simulink model "Validity"  (R2021b)
settings: Solver=FixedStepDiscrete  StartTime=0.0  StopTime=10.0  FixedStep=0.1  RelTol=1e-3  EnableMultiTasking=on
undefined symbols (not defined in the file or in its folder): sldvsubsys
libraries: sldvlib x1
settings Model: DVExtractedSubsystem=Validity  Creator=Alessandro  LastModifiedBy=Alessandro
settings SolverCC: AlgebraicLoopSolver=TrustRegion  AutoInsertRateTranBlk=on
settings DataIOCC: LimitDataPoints=on
settings OptimizationCC: LifeSpan=inf
settings DebuggingCC: FrameProcessingCompatibilityMsg=none  AllowSymbolicDim=off  SFUnexpectedBacktrackingDiag=warning  SFNoUnconditionalDefaultTransitionDiag=warning  SFExecutionAtInitializationDiag=none  ArithmeticOperatorsInVariantConditions=warning
settings SFSimCC: SimUseLocalCustomCode=off  CustomCodeUndefinedFunction=UseInterfaceOnly
settings RTWCC: RTWUseLocalCustomCode=off
settings CodeAppCC: StateflowObjectComments=on
settings GRTTargetCC: TargetLangStandard=C89/C90 (ANSI)
settings ConfigComp: CovMetricSettings=dw  CovSaveCumulativeToWorkspaceVar=on  CovSaveSingleToWorkspaceVar=on  CovExternalEMLEnable=off  CovSFcnEnable=off  DVMode=PropertyProving  DVTestSuiteOptimization=Auto  DVDetectOutOfBounds=on  DVModelReferenceHarness=on

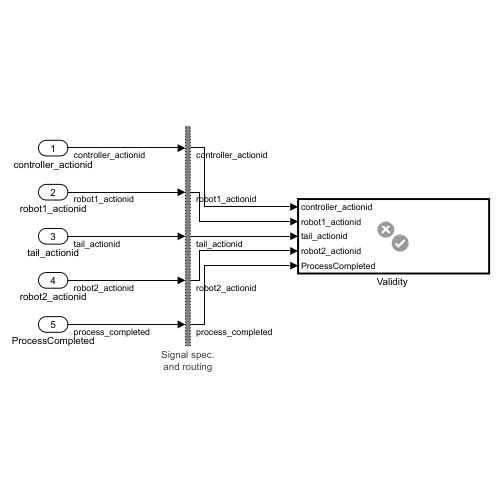
[thumbnail: Simulink's stored preview of the top-level diagram]
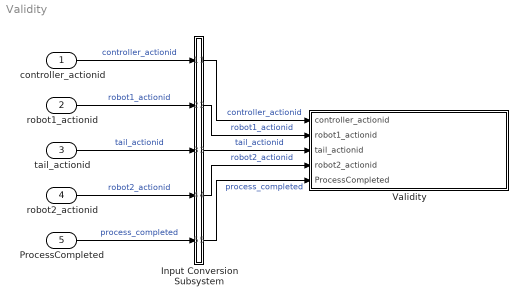
== system Validity ==
  controller_actionid : Inport  OutDataTypeStr=double  PortDimensions=[1]  SampleTime=0.1  Interpolate=off
  robot1_actionid : Inport  Port=2  OutDataTypeStr=double  PortDimensions=[1]  SampleTime=0.1  Interpolate=off
  tail_actionid : Inport  Port=3  OutDataTypeStr=double  PortDimensions=[1]  SampleTime=0.1  Interpolate=off
  robot2_actionid : Inport  Port=4  OutDataTypeStr=double  PortDimensions=[1]  SampleTime=0.1  Interpolate=off
  ProcessCompleted : Inport  Port=5  OutDataTypeStr=double  PortDimensions=[1]  SampleTime=0.1  Interpolate=off
  Input Conversion Subsystem : Subsystem  Tag=__SLT_ICS__  Description=|
      | Signal spec.
      | and routing
      settings: AttributesFormatString=%<Description>
  "Validity " : Subsystem  Tag=VerificationSubsystem  DisableCoverage=on  LoadFcn=sldvsubsys('check')  TreatAsAtomicUnit=on  SimViewingDevice=on  mask(VerificationSubsystem){}
      mask init:
      | sldvsubsys('maskInit');
      settings: CopyFcn=sldvsubsys('copy');  OpenFcn=open_system(gcb,'force');
      settings: PreSaveFcn=|
      | set_param(gcb,'SimViewingDevice','on');
      | sldvsubsys('check');
      mask Help: helpview(fullfile(docroot,'toolbox','sldv','sldv.map'),'verificationsubsystem')
      mask Display: image(imread('sldvicon_versubsys.png','BackGroundColor',[1 1 1]),'center');
  wires:
  controller_actionid/1 -> Input Conversion Subsystem/1(Inport_1)  "controller_actionid"
  robot1_actionid/1 -> Input Conversion Subsystem/2(Inport_2)  "robot1_actionid"
  tail_actionid/1 -> Input Conversion Subsystem/3(Inport_3)  "tail_actionid"
  robot2_actionid/1 -> Input Conversion Subsystem/4(Inport_4)  "robot2_actionid"
  ProcessCompleted/1 -> Input Conversion Subsystem/5(Inport_5)  "process_completed"
  Input Conversion Subsystem/1(Outport_1) -> "Validity "/1(controller_actionid)  "controller_actionid"
  Input Conversion Subsystem/2(Outport_2) -> "Validity "/2(robot1_actionid)  "robot1_actionid"
  Input Conversion Subsystem/3(Outport_3) -> "Validity "/3(tail_actionid)  "tail_actionid"
  Input Conversion Subsystem/4(Outport_4) -> "Validity "/4(robot2_actionid)  "robot2_actionid"
  Input Conversion Subsystem/5(Outport_5) -> "Validity "/5(ProcessCompleted)  "process_completed"

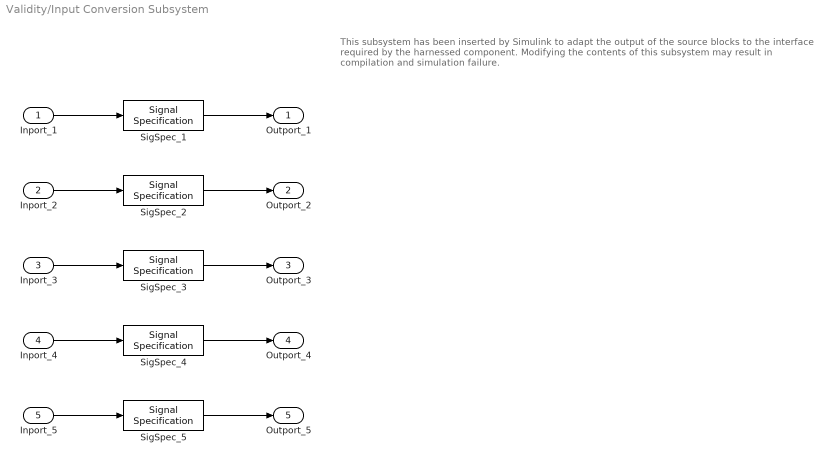
== system Validity/Input Conversion Subsystem ==
  note: This subsystem has been inserted by Simulink to adapt the output of the source blocks to the interface required by the harnessed component.
      |  Modifying the contents of this subsystem may result in compilation and simulation failure.
  Inport_1 : Inport
  Inport_2 : Inport  Port=2
  Inport_3 : Inport  Port=3
  Inport_4 : Inport  Port=4
  Inport_5 : Inport  Port=5
  SigSpec_{1..5} (5 alike) : SignalSpecification  OutDataTypeStr=double  Dimensions=[1]  SampleTime=0.1
  Outport_1 : Outport
  Outport_2 : Outport  Port=2
  Outport_3 : Outport  Port=3
  Outport_4 : Outport  Port=4
  Outport_5 : Outport  Port=5
  wires:
  SigSpec_1/1 -> Outport_1/1
  Inport_1/1 -> SigSpec_1/1
  SigSpec_2/1 -> Outport_2/1
  Inport_2/1 -> SigSpec_2/1
  SigSpec_3/1 -> Outport_3/1
  Inport_3/1 -> SigSpec_3/1
  SigSpec_4/1 -> Outport_4/1
  Inport_4/1 -> SigSpec_4/1
  SigSpec_5/1 -> Outport_5/1
  Inport_5/1 -> SigSpec_5/1

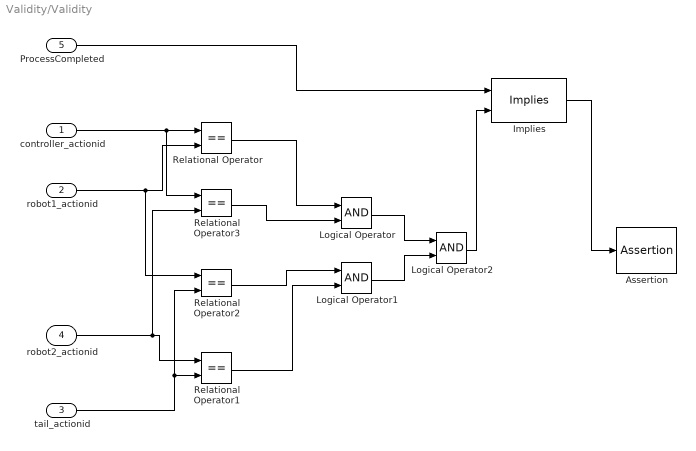
== system Validity/Validity  ==
  controller_actionid : Inport
  robot1_actionid : Inport  Port=2
  tail_actionid : Inport  Port=3
  robot2_actionid : Inport  Port=4
  ProcessCompleted : Inport  Port=5
  Assertion : Assertion
  Implies : sldvlib/Verification Utilities/Implies
      settings: SourceProductBaseCode=SL
  Logical Operator : Logic  AllPortsSameDT=off  OutDataTypeStr=boolean
  Logical Operator1 : Logic  AllPortsSameDT=off  OutDataTypeStr=boolean
  Logical Operator2 : Logic  AllPortsSameDT=off  OutDataTypeStr=boolean
  Relational Operator{,1..3} (4 alike) : RelationalOperator  Operator===  OutDataTypeStr=boolean  RndMeth=Simplest
  wires:
  Implies/1 -> Assertion/1
  ProcessCompleted/1 -> Implies/1
  Logical Operator2/1 -> Implies/2
  Logical Operator1/1 -> Logical Operator2/2
  Logical Operator/1 -> Logical Operator2/1
  Relational Operator1/1 -> Logical Operator1/2
  Relational Operator2/1 -> Logical Operator1/1
  Relational Operator3/1 -> Logical Operator/2
  Relational Operator/1 -> Logical Operator/1
  tail_actionid/1 -> Relational Operator1/2, Relational Operator2/2
  robot2_actionid/1 -> Relational Operator1/1, Relational Operator3/2
  robot1_actionid/1 -> Relational Operator/2, Relational Operator2/1
  controller_actionid/1 -> Relational Operator/1, Relational Operator3/1
